simulink model "control_project"  (R2016a)
settings: Solver=VariableStepAuto  StartTime=0.0  StopTime=10  MaxStep=0.01  RelTol=1e-4
values from neighbouring files (symbols this model uses):
  s = tf('s')    [Compensated_time_response.m]    (also in Uncompensated_time_response.m)
libraries: slctrlblks x1
settings Model: Creator=medo_  LastModifiedBy=medo_
settings DataIOCC: LimitDataPoints=on  SaveOutput=off  SaveTime=off
settings OptimizationCC: ExpressionDepthLimit=2147483647  LifeSpan=1
settings DebuggingCC: UnderspecifiedInitializationDetection=Classic  MergeDetectMultiDrivingBlocksExec=none  FcnCallInpInsideContextMsg=EnableAllAsWarning  AllowSymbolicDim=off  StateNameClashWarn=warning
settings GRTTargetCC: CombineOutputUpdateFcns=off  GRTInterface=on

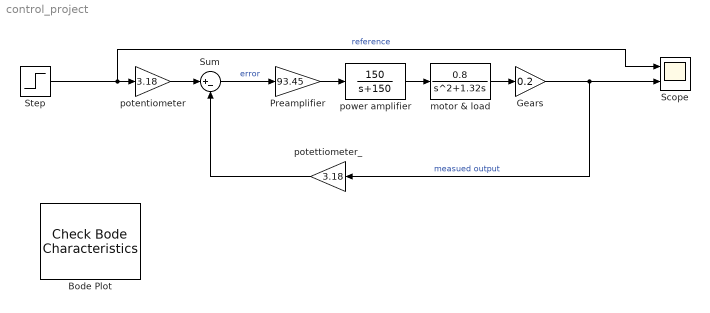
== system control_project ==
  Bode Plot : slctrlblks/Model Verification/Check Bode  Characteristics  InstantiateOnLoad=on  SaveOperatingPoints=off  LinearizationIOs={}  LinearizeAt=SnapshotTimes  SnapshotTimes=[0]  TriggerType=rising  SampleTime=auto  RateConversionMethod=zoh  PreWarpFreq=10  UseExactDelayModel=off  UseFullBlockNameLabels=off  UseBusSignalLabels=off  enabled=on  stopWhenAssertionFail=off  export=off  ViewDlgPos=[114.6 247.4 509.6 389.6]  OpenViewOnLoad=off  LaunchViewOnOpen=off  FrequencyUnits=rad/s  MagnitudeUnits=dB  PhaseUnits=deg  TimeUnits=seconds  EnableUpperBound=off  UpperBoundFrequencies=[]  UpperBoundMagnitudes=[]  EnableLowerBound=off  LowerBoundFrequencies=[]  LowerBoundMagnitudes=[]
  Gears : Gain  Gain=0.2
  Preamplifier : Gain  Gain=93.45
  Scope : Scope  NumInputPorts=2
  Step : Step  SampleTime=0
  Sum : Sum  Inputs=|+-
  motor & load : TransferFcn  Numerator=[0.8]  Denominator=[1 1.32 0]
  potentiometer : Gain  Gain=3.18
  potettiometer_ : Gain  Gain=3.18
  power amplifier : TransferFcn  Numerator=[150]  Denominator=[1 150]
  wires:
  Gears/1 -> Scope/2, potettiometer_/1  "measued output"
  Sum/1 -> Preamplifier/1  "error"
  power amplifier/1 -> motor & load/1
  motor & load/1 -> Gears/1
  Preamplifier/1 -> power amplifier/1
  potentiometer/1 -> Sum/1
  Step/1 -> Scope/1, potentiometer/1  "reference"
  potettiometer_/1 -> Sum/2
